simulink model "jacobian_test_sim"  (R2018b)
settings: Solver=VariableStepAuto  StartTime=0.0  StopTime=10.0  RelTol=1e-3
undefined symbols (not defined in the file): g, Ixx, m, x0
settings Model: Creator=longh  LastModifiedBy=arthus

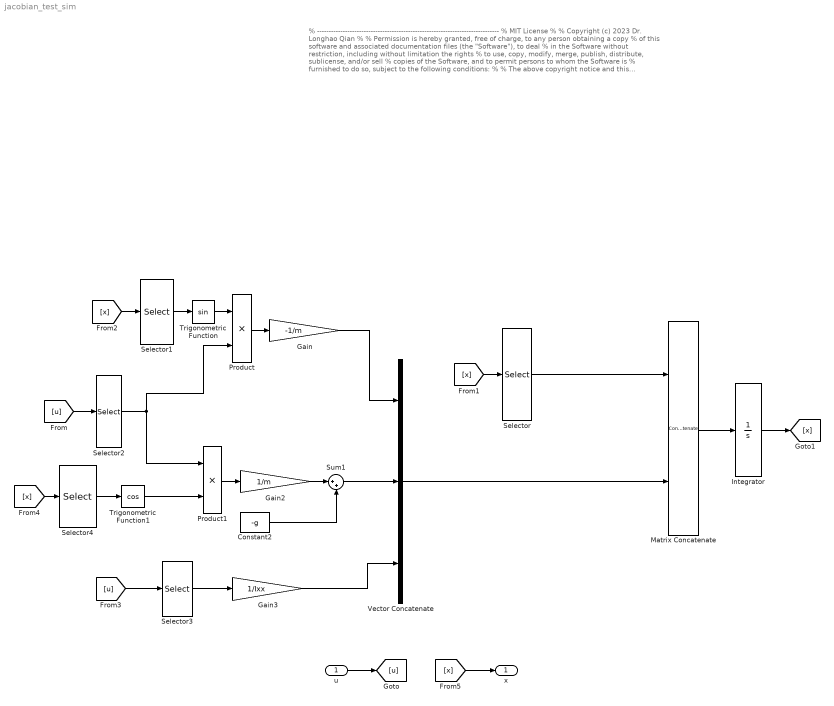
== system jacobian_test_sim ==
  note: % ------------------------------------------------------------------------------
      | % MIT License
      | %
      | % Copyright (c) 2023 Dr. Longhao Qian
      | %
      | % Permission is hereby granted, free of charge, to any person obtaining a copy
      | % of this software and associated documentation files (the "Software"), to deal
      | % in the Software without restriction, including without limitation the rights
      | % to use, copy, modify, merge, publish, distribute, sublicense, and/or sell
      | % copies of the Software, and to permit persons to whom the Software is
      | % furnished to do so, subject to the following conditions:
      | %
      | % The above copyright notice and this permission notice shall be included in all
      | % copies or substantial portions of the Software.
      | %
      | % THE SOFTWARE IS PROVIDED "AS IS", WITHOUT WARRANTY OF ANY KIND, EXPRESS OR
      | % IMPLIED, INCLUDING BUT NOT LIMITED TO THE WARRANTIES OF MERCHANTABILITY,
      | % FITNESS FOR A PARTICULAR PURPOSE AND NONINFRINGEMENT. IN NO EVENT SHALL THE
      | % AUTHORS OR COPYRIGHT HOLDERS BE LIABLE FOR ANY CLAIM, DAMAGES OR OTHER
      | % LIABILITY, WHETHER IN AN ACTION OF CONTRACT, TORT OR OTHERWISE, ARISING FROM,
      | % OUT OF OR IN CONNECTION WITH THE SOFTWARE OR THE USE OR OTHER DEALINGS IN THE
      | % SOFTWARE.
      | % ------------------------------------------------------------------------------
  u : Inport
  Constant2 : Constant  Value=-g
  Gain : Gain  Gain=-1/m
  Gain2 : Gain  Gain=1/m
  Gain3 : Gain  Gain=1/Ixx
  Integrator : Integrator  InitialCondition=x0
  Matrix Concatenate : Concatenate  Mode=Multidimensional array
  Product : Product
  Product1 : Product
  Selector : Selector  InputPortWidth=6  IndexOptions=Index vector (dialog)  Indices=[4 5 6]  OutputSizes=1
  Selector1 : Selector  InputPortWidth=6  IndexOptions=Index vector (dialog)  Indices=[3]  OutputSizes=1
  Selector2 : Selector  InputPortWidth=2  IndexOptions=Index vector (dialog)  Indices=[1]  OutputSizes=1
  Selector3 : Selector  InputPortWidth=2  IndexOptions=Index vector (dialog)  Indices=[2]  OutputSizes=1
  Selector4 : Selector  InputPortWidth=6  IndexOptions=Index vector (dialog)  Indices=[3]  OutputSizes=1
  Sum1 : Sum  Inputs=|++
  Trigonometric Function : Trigonometry
  Trigonometric Function1 : Trigonometry  Operator=cos
  Vector Concatenate : Concatenate  NumInputs=3  Mode=Multidimensional array
  x : Outport
  wires:
  Integrator/1 -> [x]
  Matrix Concatenate/1 -> Integrator/1
  Vector Concatenate/1 -> Matrix Concatenate/2
  Gain/1 -> Vector Concatenate/1
  Product/1 -> Gain/1
  Trigonometric Function/1 -> Product/1
  Selector1/1 -> Trigonometric Function/1
  u/1 -> [u]
  [x] -> Selector/1
  [u] -> Selector2/1
  Selector2/1 -> Product1/1, Product/2
  [x] -> Selector1/1
  Constant2/1 -> Sum1/2
  Gain2/1 -> Sum1/1
  Sum1/1 -> Vector Concatenate/2
  [u] -> Selector3/1
  Gain3/1 -> Vector Concatenate/3
  Selector3/1 -> Gain3/1
  [x] -> Selector4/1
  Selector4/1 -> Trigonometric Function1/1
  Product1/1 -> Gain2/1
  Trigonometric Function1/1 -> Product1/2
  Selector/1 -> Matrix Concatenate/1
  [x] -> x/1
